simulink model "TST_DrvDem_SelectParameter"  (R2016b)
settings: Solver=FixedStepDiscrete  StartTime=0.0  StopTime=simTime  FixedStep=sampleTime  RelTol=1e-3
values from neighbouring files (symbols this model uses):
  testCase = 1    [initTST_DrvDem_SelectParameter_001.m]    (also in initTST_DrvDem_SelectParameter_002.m = 2; initTST_DrvDem_SelectParameter_003.m = 3)
libraries: simulink x82, UnitTest_Lib x78
(part 2 of 3)

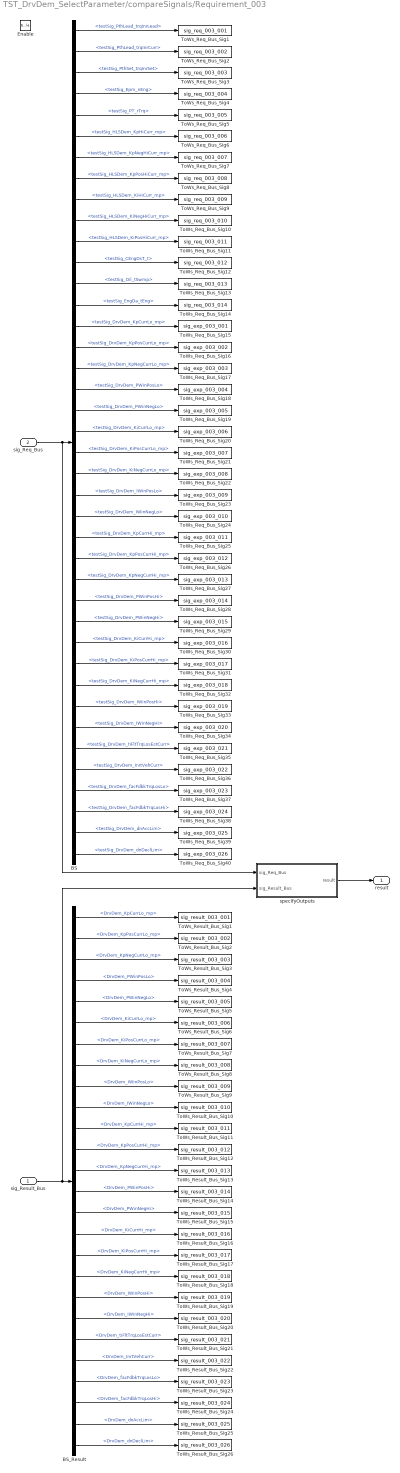
== system TST_DrvDem_SelectParameter/compareSignals/Requirement_003 ==
  sig_Result_Bus : Inport
  sig_Req_Bus : Inport  Port=2
  Enable : EnablePort
  BS : BusSelector  OutputSignals=testSig_PthLead_trqInrLead,testSig_PthLead_trqInrCurr,testSig_PthSet_trqInrSet,testSig_Epm_nEng,testSig_PT_rTrq,testSig_HLSDem_KpHiCurr_mp,testSig_HLSDem_KpNegHiCurr_mp,testSig_HLSDem_KpPosHiCurr_mp,testSig_HLSDem_KiHiCurr_mp,testSig_HLSDem_KiNegHiCurr_mp,testSig_HLSDem_KiPosHiCurr_mp,testSig_CEngDsT_t,testSig_Oil_tSwmp,testSig_EngDa_tEng,testSig_DrvDem_KpCurrLo_mp,testSig_DrvDem_KpPosCurrLo_mp,testSig_DrvDem_KpNegCurrLo_mp,testSig_DrvDem_PWinPosLo,testSig_DrvDem_PWinNegLo,testSig_DrvDem_KiCurrLo_mp,testSig_DrvDem_KiPosCurrLo_mp,testSig_DrvDem_KiNegCurrLo_mp,testSig_DrvDem_IWinPosLo,testSig_DrvDem_IWinNegLo,testSig_DrvDem_KpCurrHi_mp,testSig_DrvDem_KpPosCurrHi_mp,testSig_DrvDem_KpNegCurrHi_mp,testSig_DrvDem_PWinPosHi,testSig_DrvDem_PWinNegHi,testSig_DrvDem_KiCurrHi_mp,testSig_DrvDem_KiPosCurrHi_mp,testSig_DrvDem_KiNegCurrHi_mp,testSig_DrvDem_IWinPosHi,testSig_DrvDem_IWinNegHi,testSig_DrvDem_tiFltTrqLosEstCurr,testSig_DrvDem_InrtVehCurr,testSig_DrvDem_facFdbkTrqLosLo,testSig_DrvDem_facFdbkTrqLosHi,testSig_DrvDem_dnAccLim,testSig_DrvDem_dnDeclLim
  BS_Result : BusSelector  OutputSignals=DrvDem_KpCurrLo_mp,DrvDem_KpPosCurrLo_mp,DrvDem_KpNegCurrLo_mp,DrvDem_PWinPosLo,DrvDem_PWinNegLo,DrvDem_KiCurrLo_mp,DrvDem_KiPosCurrLo_mp,DrvDem_KiNegCurrLo_mp,DrvDem_IWinPosLo,DrvDem_IWinNegLo,DrvDem_KpCurrHi_mp,DrvDem_KpPosCurrHi_mp,DrvDem_KpNegCurrHi_mp,DrvDem_PWinPosHi,DrvDem_PWinNegHi,DrvDem_KiCurrHi_mp,DrvDem_KiPosCurrHi_mp,DrvDem_KiNegCurrHi_mp,DrvDem_IWinPosHi,DrvDem_IWinNegHi,DrvDem_tiFltTrqLosEstCurr,DrvDem_InrtVehCurr,DrvDem_facFdbkTrqLosLo,DrvDem_facFdbkTrqLosHi,DrvDem_dnAccLim,DrvDem_dnDeclLim
  ToWs_Req_Bus_Sig1 : ToWorkspace  VariableName=sig_req_003_001  SaveFormat=Structure With Time
  ToWs_Req_Bus_Sig10 : ToWorkspace  VariableName=sig_req_003_010  SaveFormat=Structure With Time
  ToWs_Req_Bus_Sig11 : ToWorkspace  VariableName=sig_req_003_011  SaveFormat=Structure With Time
  ToWs_Req_Bus_Sig12 : ToWorkspace  VariableName=sig_req_003_012  SaveFormat=Structure With Time
  ToWs_Req_Bus_Sig13 : ToWorkspace  VariableName=sig_req_003_013  SaveFormat=Structure With Time
  ToWs_Req_Bus_Sig14 : ToWorkspace  VariableName=sig_req_003_014  SaveFormat=Structure With Time
  ToWs_Req_Bus_Sig15 : ToWorkspace  VariableName=sig_exp_003_001  SaveFormat=Structure With Time
  ToWs_Req_Bus_Sig16 : ToWorkspace  VariableName=sig_exp_003_002  SaveFormat=Structure With Time
  ToWs_Req_Bus_Sig17 : ToWorkspace  VariableName=sig_exp_003_003  SaveFormat=Structure With Time
  ToWs_Req_Bus_Sig18 : ToWorkspace  VariableName=sig_exp_003_004  SaveFormat=Structure With Time
  ToWs_Req_Bus_Sig19 : ToWorkspace  VariableName=sig_exp_003_005  SaveFormat=Structure With Time
  ToWs_Req_Bus_Sig2 : ToWorkspace  VariableName=sig_req_003_002  SaveFormat=Structure With Time
  ToWs_Req_Bus_Sig20 : ToWorkspace  VariableName=sig_exp_003_006  SaveFormat=Structure With Time
  ToWs_Req_Bus_Sig21 : ToWorkspace  VariableName=sig_exp_003_007  SaveFormat=Structure With Time
  ToWs_Req_Bus_Sig22 : ToWorkspace  VariableName=sig_exp_003_008  SaveFormat=Structure With Time
  ToWs_Req_Bus_Sig23 : ToWorkspace  VariableName=sig_exp_003_009  SaveFormat=Structure With Time
  ToWs_Req_Bus_Sig24 : ToWorkspace  VariableName=sig_exp_003_010  SaveFormat=Structure With Time
  ToWs_Req_Bus_Sig25 : ToWorkspace  VariableName=sig_exp_003_011  SaveFormat=Structure With Time
  ToWs_Req_Bus_Sig26 : ToWorkspace  VariableName=sig_exp_003_012  SaveFormat=Structure With Time
  ToWs_Req_Bus_Sig27 : ToWorkspace  VariableName=sig_exp_003_013  SaveFormat=Structure With Time
  ToWs_Req_Bus_Sig28 : ToWorkspace  VariableName=sig_exp_003_014  SaveFormat=Structure With Time
  ToWs_Req_Bus_Sig29 : ToWorkspace  VariableName=sig_exp_003_015  SaveFormat=Structure With Time
  ToWs_Req_Bus_Sig3 : ToWorkspace  VariableName=sig_req_003_003  SaveFormat=Structure With Time
  ToWs_Req_Bus_Sig30 : ToWorkspace  VariableName=sig_exp_003_016  SaveFormat=Structure With Time
  ToWs_Req_Bus_Sig31 : ToWorkspace  VariableName=sig_exp_003_017  SaveFormat=Structure With Time
  ToWs_Req_Bus_Sig32 : ToWorkspace  VariableName=sig_exp_003_018  SaveFormat=Structure With Time
  ToWs_Req_Bus_Sig33 : ToWorkspace  VariableName=sig_exp_003_019  SaveFormat=Structure With Time
  ToWs_Req_Bus_Sig34 : ToWorkspace  VariableName=sig_exp_003_020  SaveFormat=Structure With Time
  ToWs_Req_Bus_Sig35 : ToWorkspace  VariableName=sig_exp_003_021  SaveFormat=Structure With Time
  ToWs_Req_Bus_Sig36 : ToWorkspace  VariableName=sig_exp_003_022  SaveFormat=Structure With Time
  ToWs_Req_Bus_Sig37 : ToWorkspace  VariableName=sig_exp_003_023  SaveFormat=Structure With Time
  ToWs_Req_Bus_Sig38 : ToWorkspace  VariableName=sig_exp_003_024  SaveFormat=Structure With Time
  ToWs_Req_Bus_Sig39 : ToWorkspace  VariableName=sig_exp_003_025  SaveFormat=Structure With Time
  ToWs_Req_Bus_Sig4 : ToWorkspace  VariableName=sig_req_003_004  SaveFormat=Structure With Time
  ToWs_Req_Bus_Sig40 : ToWorkspace  VariableName=sig_exp_003_026  SaveFormat=Structure With Time
  ToWs_Req_Bus_Sig5 : ToWorkspace  VariableName=sig_req_003_005  SaveFormat=Structure With Time
  ToWs_Req_Bus_Sig6 : ToWorkspace  VariableName=sig_req_003_006  SaveFormat=Structure With Time
  ToWs_Req_Bus_Sig7 : ToWorkspace  VariableName=sig_req_003_007  SaveFormat=Structure With Time
  ToWs_Req_Bus_Sig8 : ToWorkspace  VariableName=sig_req_003_008  SaveFormat=Structure With Time
  ToWs_Req_Bus_Sig9 : ToWorkspace  VariableName=sig_req_003_009  SaveFormat=Structure With Time
  ToWs_Result_Bus_Sig1 : ToWorkspace  VariableName=sig_result_003_001  SaveFormat=Structure With Time
  ToWs_Result_Bus_Sig10 : ToWorkspace  VariableName=sig_result_003_010  SaveFormat=Structure With Time
  ToWs_Result_Bus_Sig11 : ToWorkspace  VariableName=sig_result_003_011  SaveFormat=Structure With Time
  ToWs_Result_Bus_Sig12 : ToWorkspace  VariableName=sig_result_003_012  SaveFormat=Structure With Time
  ToWs_Result_Bus_Sig13 : ToWorkspace  VariableName=sig_result_003_013  SaveFormat=Structure With Time
  ToWs_Result_Bus_Sig14 : ToWorkspace  VariableName=sig_result_003_014  SaveFormat=Structure With Time
  ToWs_Result_Bus_Sig15 : ToWorkspace  VariableName=sig_result_003_015  SaveFormat=Structure With Time
  ToWs_Result_Bus_Sig16 : ToWorkspace  VariableName=sig_result_003_016  SaveFormat=Structure With Time
  ToWs_Result_Bus_Sig17 : ToWorkspace  VariableName=sig_result_003_017  SaveFormat=Structure With Time
  ToWs_Result_Bus_Sig18 : ToWorkspace  VariableName=sig_result_003_018  SaveFormat=Structure With Time
  ToWs_Result_Bus_Sig19 : ToWorkspace  VariableName=sig_result_003_019  SaveFormat=Structure With Time
  ToWs_Result_Bus_Sig2 : ToWorkspace  VariableName=sig_result_003_002  SaveFormat=Structure With Time
  ToWs_Result_Bus_Sig20 : ToWorkspace  VariableName=sig_result_003_020  SaveFormat=Structure With Time
  ToWs_Result_Bus_Sig21 : ToWorkspace  VariableName=sig_result_003_021  SaveFormat=Structure With Time
  ToWs_Result_Bus_Sig22 : ToWorkspace  VariableName=sig_result_003_022  SaveFormat=Structure With Time
  ToWs_Result_Bus_Sig23 : ToWorkspace  VariableName=sig_result_003_023  SaveFormat=Structure With Time
  ToWs_Result_Bus_Sig24 : ToWorkspace  VariableName=sig_result_003_024  SaveFormat=Structure With Time
  ToWs_Result_Bus_Sig25 : ToWorkspace  VariableName=sig_result_003_025  SaveFormat=Structure With Time
  ToWs_Result_Bus_Sig26 : ToWorkspace  VariableName=sig_result_003_026  SaveFormat=Structure With Time
  ToWs_Result_Bus_Sig3 : ToWorkspace  VariableName=sig_result_003_003  SaveFormat=Structure With Time
  ToWs_Result_Bus_Sig4 : ToWorkspace  VariableName=sig_result_003_004  SaveFormat=Structure With Time
  ToWs_Result_Bus_Sig5 : ToWorkspace  VariableName=sig_result_003_005  SaveFormat=Structure With Time
  ToWs_Result_Bus_Sig6 : ToWorkspace  VariableName=sig_result_003_006  SaveFormat=Structure With Time
  ToWs_Result_Bus_Sig7 : ToWorkspace  VariableName=sig_result_003_007  SaveFormat=Structure With Time
  ToWs_Result_Bus_Sig8 : ToWorkspace  VariableName=sig_result_003_008  SaveFormat=Structure With Time
  ToWs_Result_Bus_Sig9 : ToWorkspace  VariableName=sig_result_003_009  SaveFormat=Structure With Time
  specifyOutputs : Subsystem
  result : Outport
  wires:
  sig_Req_Bus/1 -> BS/1, specifyOutputs/1(sig_Req_Bus)
  BS/1 -> ToWs_Req_Bus_Sig1/1  "<testSig_PthLead_trqInrLead>"
  BS/2 -> ToWs_Req_Bus_Sig2/1  "<testSig_PthLead_trqInrCurr>"
  BS/3 -> ToWs_Req_Bus_Sig3/1  "<testSig_PthSet_trqInrSet>"
  BS/4 -> ToWs_Req_Bus_Sig4/1  "<testSig_Epm_nEng>"
  BS/5 -> ToWs_Req_Bus_Sig5/1  "<testSig_PT_rTrq>"
  BS/6 -> ToWs_Req_Bus_Sig6/1  "<testSig_HLSDem_KpHiCurr_mp>"
  BS/7 -> ToWs_Req_Bus_Sig7/1  "<testSig_HLSDem_KpNegHiCurr_mp>"
  BS/8 -> ToWs_Req_Bus_Sig8/1  "<testSig_HLSDem_KpPosHiCurr_mp>"
  BS/9 -> ToWs_Req_Bus_Sig9/1  "<testSig_HLSDem_KiHiCurr_mp>"
  BS/10 -> ToWs_Req_Bus_Sig10/1  "<testSig_HLSDem_KiNegHiCurr_mp>"
  BS/11 -> ToWs_Req_Bus_Sig11/1  "<testSig_HLSDem_KiPosHiCurr_mp>"
  BS/12 -> ToWs_Req_Bus_Sig12/1  "<testSig_CEngDsT_t>"
  BS/13 -> ToWs_Req_Bus_Sig13/1  "<testSig_Oil_tSwmp>"
  BS/14 -> ToWs_Req_Bus_Sig14/1  "<testSig_EngDa_tEng>"
  BS/15 -> ToWs_Req_Bus_Sig15/1  "<testSig_DrvDem_KpCurrLo_mp>"
  BS/16 -> ToWs_Req_Bus_Sig16/1  "<testSig_DrvDem_KpPosCurrLo_mp>"
  BS/17 -> ToWs_Req_Bus_Sig17/1  "<testSig_DrvDem_KpNegCurrLo_mp>"
  BS/18 -> ToWs_Req_Bus_Sig18/1  "<testSig_DrvDem_PWinPosLo>"
  BS/19 -> ToWs_Req_Bus_Sig19/1  "<testSig_DrvDem_PWinNegLo>"
  BS/20 -> ToWs_Req_Bus_Sig20/1  "<testSig_DrvDem_KiCurrLo_mp>"
  BS/21 -> ToWs_Req_Bus_Sig21/1  "<testSig_DrvDem_KiPosCurrLo_mp>"
  BS/22 -> ToWs_Req_Bus_Sig22/1  "<testSig_DrvDem_KiNegCurrLo_mp>"
  BS/23 -> ToWs_Req_Bus_Sig23/1  "<testSig_DrvDem_IWinPosLo>"
  BS/24 -> ToWs_Req_Bus_Sig24/1  "<testSig_DrvDem_IWinNegLo>"
  BS/25 -> ToWs_Req_Bus_Sig25/1  "<testSig_DrvDem_KpCurrHi_mp>"
  BS/26 -> ToWs_Req_Bus_Sig26/1  "<testSig_DrvDem_KpPosCurrHi_mp>"
  BS/27 -> ToWs_Req_Bus_Sig27/1  "<testSig_DrvDem_KpNegCurrHi_mp>"
  BS/28 -> ToWs_Req_Bus_Sig28/1  "<testSig_DrvDem_PWinPosHi>"
  BS/29 -> ToWs_Req_Bus_Sig29/1  "<testSig_DrvDem_PWinNegHi>"
  BS/30 -> ToWs_Req_Bus_Sig30/1  "<testSig_DrvDem_KiCurrHi_mp>"
  BS/31 -> ToWs_Req_Bus_Sig31/1  "<testSig_DrvDem_KiPosCurrHi_mp>"
  BS/32 -> ToWs_Req_Bus_Sig32/1  "<testSig_DrvDem_KiNegCurrHi_mp>"
  BS/33 -> ToWs_Req_Bus_Sig33/1  "<testSig_DrvDem_IWinPosHi>"
  BS/34 -> ToWs_Req_Bus_Sig34/1  "<testSig_DrvDem_IWinNegHi>"
  BS/35 -> ToWs_Req_Bus_Sig35/1  "<testSig_DrvDem_tiFltTrqLosEstCurr>"
  BS/36 -> ToWs_Req_Bus_Sig36/1  "<testSig_DrvDem_InrtVehCurr>"
  BS/37 -> ToWs_Req_Bus_Sig37/1  "<testSig_DrvDem_facFdbkTrqLosLo>"
  BS/38 -> ToWs_Req_Bus_Sig38/1  "<testSig_DrvDem_facFdbkTrqLosHi>"
  BS/39 -> ToWs_Req_Bus_Sig39/1  "<testSig_DrvDem_dnAccLim>"
  BS/40 -> ToWs_Req_Bus_Sig40/1  "<testSig_DrvDem_dnDeclLim>"
  sig_Result_Bus/1 -> BS_Result/1, specifyOutputs/2(sig_Result_Bus)
  BS_Result/1 -> ToWs_Result_Bus_Sig1/1  "<DrvDem_KpCurrLo_mp>"
  BS_Result/2 -> ToWs_Result_Bus_Sig2/1  "<DrvDem_KpPosCurrLo_mp>"
  BS_Result/3 -> ToWs_Result_Bus_Sig3/1  "<DrvDem_KpNegCurrLo_mp>"
  BS_Result/4 -> ToWs_Result_Bus_Sig4/1  "<DrvDem_PWinPosLo>"
  BS_Result/5 -> ToWs_Result_Bus_Sig5/1  "<DrvDem_PWinNegLo>"
  BS_Result/6 -> ToWs_Result_Bus_Sig6/1  "<DrvDem_KiCurrLo_mp>"
  BS_Result/7 -> ToWs_Result_Bus_Sig7/1  "<DrvDem_KiPosCurrLo_mp>"
  BS_Result/8 -> ToWs_Result_Bus_Sig8/1  "<DrvDem_KiNegCurrLo_mp>"
  BS_Result/9 -> ToWs_Result_Bus_Sig9/1  "<DrvDem_IWinPosLo>"
  BS_Result/10 -> ToWs_Result_Bus_Sig10/1  "<DrvDem_IWinNegLo>"
  BS_Result/11 -> ToWs_Result_Bus_Sig11/1  "<DrvDem_KpCurrHi_mp>"
  BS_Result/12 -> ToWs_Result_Bus_Sig12/1  "<DrvDem_KpPosCurrHi_mp>"
  BS_Result/13 -> ToWs_Result_Bus_Sig13/1  "<DrvDem_KpNegCurrHi_mp>"
  BS_Result/14 -> ToWs_Result_Bus_Sig14/1  "<DrvDem_PWinPosHi>"
  BS_Result/15 -> ToWs_Result_Bus_Sig15/1  "<DrvDem_PWinNegHi>"
  BS_Result/16 -> ToWs_Result_Bus_Sig16/1  "<DrvDem_KiCurrHi_mp>"
  BS_Result/17 -> ToWs_Result_Bus_Sig17/1  "<DrvDem_KiPosCurrHi_mp>"
  BS_Result/18 -> ToWs_Result_Bus_Sig18/1  "<DrvDem_KiNegCurrHi_mp>"
  BS_Result/19 -> ToWs_Result_Bus_Sig19/1  "<DrvDem_IWinPosHi>"
  BS_Result/20 -> ToWs_Result_Bus_Sig20/1  "<DrvDem_IWinNegHi>"
  BS_Result/21 -> ToWs_Result_Bus_Sig21/1  "<DrvDem_tiFltTrqLosEstCurr>"
  BS_Result/22 -> ToWs_Result_Bus_Sig22/1  "<DrvDem_InrtVehCurr>"
  BS_Result/23 -> ToWs_Result_Bus_Sig23/1  "<DrvDem_facFdbkTrqLosLo>"
  BS_Result/24 -> ToWs_Result_Bus_Sig24/1  "<DrvDem_facFdbkTrqLosHi>"
  BS_Result/25 -> ToWs_Result_Bus_Sig25/1  "<DrvDem_dnAccLim>"
  BS_Result/26 -> ToWs_Result_Bus_Sig26/1  "<DrvDem_dnDeclLim>"
  specifyOutputs/1(result) -> result/1

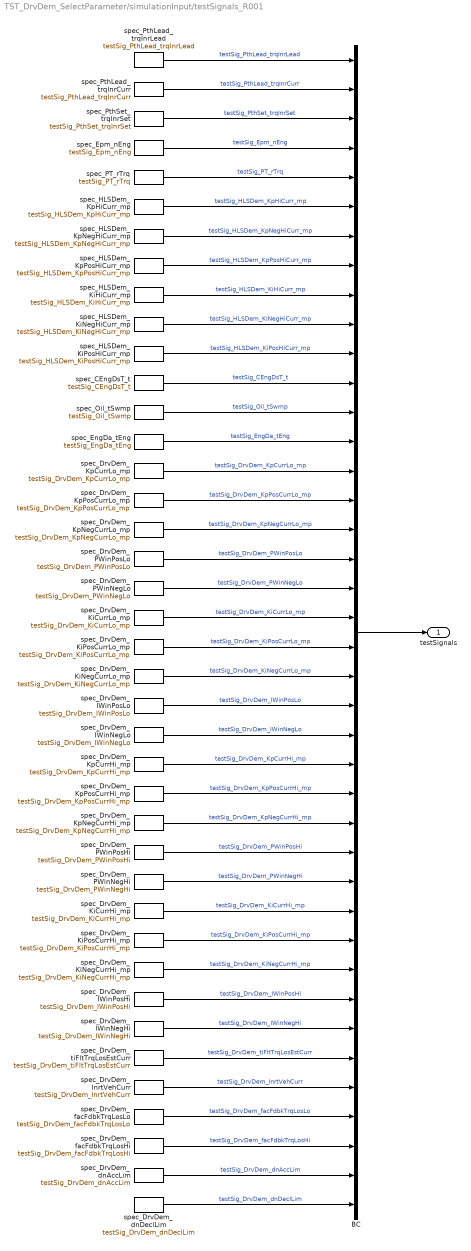
== system TST_DrvDem_SelectParameter/simulationInput/testSignals_R001 ==
  BC : BusCreator  Inputs=40
  spec_CEngDsT_t : FromWorkspace  VariableName=testSig_CEngDsT_t  Interpolate=off  OutputAfterFinalValue=Holding final value
  spec_DrvDem_IWinNegHi : FromWorkspace  VariableName=testSig_DrvDem_IWinNegHi  Interpolate=off  OutputAfterFinalValue=Holding final value
  spec_DrvDem_IWinNegLo : FromWorkspace  VariableName=testSig_DrvDem_IWinNegLo  Interpolate=off  OutputAfterFinalValue=Holding final value
  spec_DrvDem_IWinPosHi : FromWorkspace  VariableName=testSig_DrvDem_IWinPosHi  Interpolate=off  OutputAfterFinalValue=Holding final value
  spec_DrvDem_IWinPosLo : FromWorkspace  VariableName=testSig_DrvDem_IWinPosLo  Interpolate=off  OutputAfterFinalValue=Holding final value
  spec_DrvDem_InrtVehCurr : FromWorkspace  VariableName=testSig_DrvDem_InrtVehCurr  Interpolate=off  OutputAfterFinalValue=Holding final value
  spec_DrvDem_KiCurrHi_mp : FromWorkspace  VariableName=testSig_DrvDem_KiCurrHi_mp  Interpolate=off  OutputAfterFinalValue=Holding final value
  spec_DrvDem_KiCurrLo_mp : FromWorkspace  VariableName=testSig_DrvDem_KiCurrLo_mp  Interpolate=off  OutputAfterFinalValue=Holding final value
  spec_DrvDem_KiNegCurrHi_mp : FromWorkspace  VariableName=testSig_DrvDem_KiNegCurrHi_mp  Interpolate=off  OutputAfterFinalValue=Holding final value
  spec_DrvDem_KiNegCurrLo_mp : FromWorkspace  VariableName=testSig_DrvDem_KiNegCurrLo_mp  Interpolate=off  OutputAfterFinalValue=Holding final value
  spec_DrvDem_KiPosCurrHi_mp : FromWorkspace  VariableName=testSig_DrvDem_KiPosCurrHi_mp  Interpolate=off  OutputAfterFinalValue=Holding final value
  spec_DrvDem_KiPosCurrLo_mp : FromWorkspace  VariableName=testSig_DrvDem_KiPosCurrLo_mp  Interpolate=off  OutputAfterFinalValue=Holding final value
  spec_DrvDem_KpCurrHi_mp : FromWorkspace  VariableName=testSig_DrvDem_KpCurrHi_mp  Interpolate=off  OutputAfterFinalValue=Holding final value
  spec_DrvDem_KpCurrLo_mp : FromWorkspace  VariableName=testSig_DrvDem_KpCurrLo_mp  Interpolate=off  OutputAfterFinalValue=Holding final value
  spec_DrvDem_KpNegCurrHi_mp : FromWorkspace  VariableName=testSig_DrvDem_KpNegCurrHi_mp  Interpolate=off  OutputAfterFinalValue=Holding final value
  spec_DrvDem_KpNegCurrLo_mp : FromWorkspace  VariableName=testSig_DrvDem_KpNegCurrLo_mp  Interpolate=off  OutputAfterFinalValue=Holding final value
  spec_DrvDem_KpPosCurrHi_mp : FromWorkspace  VariableName=testSig_DrvDem_KpPosCurrHi_mp  Interpolate=off  OutputAfterFinalValue=Holding final value
  spec_DrvDem_KpPosCurrLo_mp : FromWorkspace  VariableName=testSig_DrvDem_KpPosCurrLo_mp  Interpolate=off  OutputAfterFinalValue=Holding final value
  spec_DrvDem_PWinNegHi : FromWorkspace  VariableName=testSig_DrvDem_PWinNegHi  Interpolate=off  OutputAfterFinalValue=Holding final value
  spec_DrvDem_PWinNegLo : FromWorkspace  VariableName=testSig_DrvDem_PWinNegLo  Interpolate=off  OutputAfterFinalValue=Holding final value
  spec_DrvDem_PWinPosHi : FromWorkspace  VariableName=testSig_DrvDem_PWinPosHi  Interpolate=off  OutputAfterFinalValue=Holding final value
  spec_DrvDem_PWinPosLo : FromWorkspace  VariableName=testSig_DrvDem_PWinPosLo  Interpolate=off  OutputAfterFinalValue=Holding final value
  spec_DrvDem_dnAccLim : FromWorkspace  VariableName=testSig_DrvDem_dnAccLim  Interpolate=off  OutputAfterFinalValue=Holding final value
  spec_DrvDem_dnDeclLim : FromWorkspace  VariableName=testSig_DrvDem_dnDeclLim  Interpolate=off  OutputAfterFinalValue=Holding final value
  spec_DrvDem_facFdbkTrqLosHi : FromWorkspace  VariableName=testSig_DrvDem_facFdbkTrqLosHi  Interpolate=off  OutputAfterFinalValue=Holding final value
  spec_DrvDem_facFdbkTrqLosLo : FromWorkspace  VariableName=testSig_DrvDem_facFdbkTrqLosLo  Interpolate=off  OutputAfterFinalValue=Holding final value
  spec_DrvDem_tiFltTrqLosEstCurr : FromWorkspace  VariableName=testSig_DrvDem_tiFltTrqLosEstCurr  Interpolate=off  OutputAfterFinalValue=Holding final value
  spec_EngDa_tEng : FromWorkspace  VariableName=testSig_EngDa_tEng  Interpolate=off  OutputAfterFinalValue=Holding final value
  spec_Epm_nEng : FromWorkspace  VariableName=testSig_Epm_nEng  Interpolate=off  OutputAfterFinalValue=Holding final value
  spec_HLSDem_KiHiCurr_mp : FromWorkspace  VariableName=testSig_HLSDem_KiHiCurr_mp  Interpolate=off  OutputAfterFinalValue=Holding final value
  spec_HLSDem_KiNegHiCurr_mp : FromWorkspace  VariableName=testSig_HLSDem_KiNegHiCurr_mp  Interpolate=off  OutputAfterFinalValue=Holding final value
  spec_HLSDem_KiPosHiCurr_mp : FromWorkspace  VariableName=testSig_HLSDem_KiPosHiCurr_mp  Interpolate=off  OutputAfterFinalValue=Holding final value
  spec_HLSDem_KpHiCurr_mp : FromWorkspace  VariableName=testSig_HLSDem_KpHiCurr_mp  Interpolate=off  OutputAfterFinalValue=Holding final value
  spec_HLSDem_KpNegHiCurr_mp : FromWorkspace  VariableName=testSig_HLSDem_KpNegHiCurr_mp  Interpolate=off  OutputAfterFinalValue=Holding final value
  spec_HLSDem_KpPosHiCurr_mp : FromWorkspace  VariableName=testSig_HLSDem_KpPosHiCurr_mp  Interpolate=off  OutputAfterFinalValue=Holding final value
  spec_Oil_tSwmp : FromWorkspace  VariableName=testSig_Oil_tSwmp  Interpolate=off  OutputAfterFinalValue=Holding final value
  spec_PT_rTrq : FromWorkspace  VariableName=testSig_PT_rTrq  Interpolate=off  OutputAfterFinalValue=Holding final value
  spec_PthLead_trqInrCurr : FromWorkspace  VariableName=testSig_PthLead_trqInrCurr  Interpolate=off  OutputAfterFinalValue=Holding final value
  spec_PthLead_trqInrLead : FromWorkspace  VariableName=testSig_PthLead_trqInrLead  Interpolate=off  OutputAfterFinalValue=Holding final value
  spec_PthSet_trqInrSet : FromWorkspace  VariableName=testSig_PthSet_trqInrSet  Interpolate=off  OutputAfterFinalValue=Holding final value
  testSignals : Outport
  wires:
  BC/1 -> testSignals/1
  spec_PthLead_trqInrLead/1 -> BC/1  "testSig_PthLead_trqInrLead"
  spec_PthLead_trqInrCurr/1 -> BC/2  "testSig_PthLead_trqInrCurr"
  spec_PthSet_trqInrSet/1 -> BC/3  "testSig_PthSet_trqInrSet"
  spec_Epm_nEng/1 -> BC/4  "testSig_Epm_nEng"
  spec_PT_rTrq/1 -> BC/5  "testSig_PT_rTrq"
  spec_HLSDem_KpHiCurr_mp/1 -> BC/6  "testSig_HLSDem_KpHiCurr_mp"
  spec_HLSDem_KpNegHiCurr_mp/1 -> BC/7  "testSig_HLSDem_KpNegHiCurr_mp"
  spec_HLSDem_KpPosHiCurr_mp/1 -> BC/8  "testSig_HLSDem_KpPosHiCurr_mp"
  spec_HLSDem_KiHiCurr_mp/1 -> BC/9  "testSig_HLSDem_KiHiCurr_mp"
  spec_HLSDem_KiNegHiCurr_mp/1 -> BC/10  "testSig_HLSDem_KiNegHiCurr_mp"
  spec_HLSDem_KiPosHiCurr_mp/1 -> BC/11  "testSig_HLSDem_KiPosHiCurr_mp"
  spec_CEngDsT_t/1 -> BC/12  "testSig_CEngDsT_t"
  spec_Oil_tSwmp/1 -> BC/13  "testSig_Oil_tSwmp"
  spec_EngDa_tEng/1 -> BC/14  "testSig_EngDa_tEng"
  spec_DrvDem_KpCurrLo_mp/1 -> BC/15  "testSig_DrvDem_KpCurrLo_mp"
  spec_DrvDem_KpPosCurrLo_mp/1 -> BC/16  "testSig_DrvDem_KpPosCurrLo_mp"
  spec_DrvDem_KpNegCurrLo_mp/1 -> BC/17  "testSig_DrvDem_KpNegCurrLo_mp"
  spec_DrvDem_PWinPosLo/1 -> BC/18  "testSig_DrvDem_PWinPosLo"
  spec_DrvDem_PWinNegLo/1 -> BC/19  "testSig_DrvDem_PWinNegLo"
  spec_DrvDem_KiCurrLo_mp/1 -> BC/20  "testSig_DrvDem_KiCurrLo_mp"
  spec_DrvDem_KiPosCurrLo_mp/1 -> BC/21  "testSig_DrvDem_KiPosCurrLo_mp"
  spec_DrvDem_KiNegCurrLo_mp/1 -> BC/22  "testSig_DrvDem_KiNegCurrLo_mp"
  spec_DrvDem_IWinPosLo/1 -> BC/23  "testSig_DrvDem_IWinPosLo"
  spec_DrvDem_IWinNegLo/1 -> BC/24  "testSig_DrvDem_IWinNegLo"
  spec_DrvDem_KpCurrHi_mp/1 -> BC/25  "testSig_DrvDem_KpCurrHi_mp"
  spec_DrvDem_KpPosCurrHi_mp/1 -> BC/26  "testSig_DrvDem_KpPosCurrHi_mp"
  spec_DrvDem_KpNegCurrHi_mp/1 -> BC/27  "testSig_DrvDem_KpNegCurrHi_mp"
  spec_DrvDem_PWinPosHi/1 -> BC/28  "testSig_DrvDem_PWinPosHi"
  spec_DrvDem_PWinNegHi/1 -> BC/29  "testSig_DrvDem_PWinNegHi"
  spec_DrvDem_KiCurrHi_mp/1 -> BC/30  "testSig_DrvDem_KiCurrHi_mp"
  spec_DrvDem_KiPosCurrHi_mp/1 -> BC/31  "testSig_DrvDem_KiPosCurrHi_mp"
  spec_DrvDem_KiNegCurrHi_mp/1 -> BC/32  "testSig_DrvDem_KiNegCurrHi_mp"
  spec_DrvDem_IWinPosHi/1 -> BC/33  "testSig_DrvDem_IWinPosHi"
  spec_DrvDem_IWinNegHi/1 -> BC/34  "testSig_DrvDem_IWinNegHi"
  spec_DrvDem_tiFltTrqLosEstCurr/1 -> BC/35  "testSig_DrvDem_tiFltTrqLosEstCurr"
  spec_DrvDem_InrtVehCurr/1 -> BC/36  "testSig_DrvDem_InrtVehCurr"
  spec_DrvDem_facFdbkTrqLosLo/1 -> BC/37  "testSig_DrvDem_facFdbkTrqLosLo"
  spec_DrvDem_facFdbkTrqLosHi/1 -> BC/38  "testSig_DrvDem_facFdbkTrqLosHi"
  spec_DrvDem_dnAccLim/1 -> BC/39  "testSig_DrvDem_dnAccLim"
  spec_DrvDem_dnDeclLim/1 -> BC/40  "testSig_DrvDem_dnDeclLim"

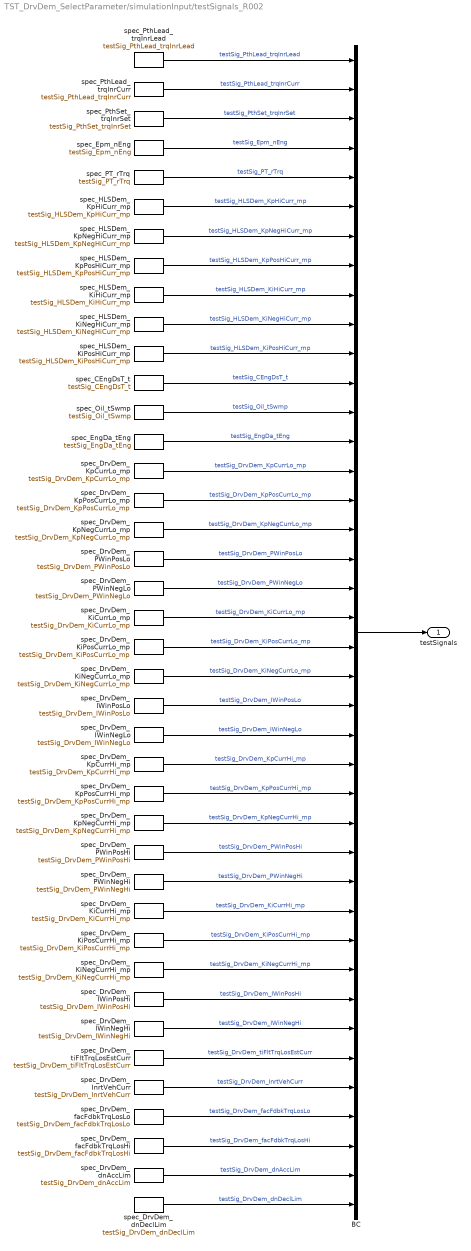
== system TST_DrvDem_SelectParameter/simulationInput/testSignals_R002 ==
  BC : BusCreator  Inputs=40
  spec_CEngDsT_t : FromWorkspace  VariableName=testSig_CEngDsT_t  Interpolate=off  OutputAfterFinalValue=Holding final value
  spec_DrvDem_IWinNegHi : FromWorkspace  VariableName=testSig_DrvDem_IWinNegHi  Interpolate=off  OutputAfterFinalValue=Holding final value
  spec_DrvDem_IWinNegLo : FromWorkspace  VariableName=testSig_DrvDem_IWinNegLo  Interpolate=off  OutputAfterFinalValue=Holding final value
  spec_DrvDem_IWinPosHi : FromWorkspace  VariableName=testSig_DrvDem_IWinPosHi  Interpolate=off  OutputAfterFinalValue=Holding final value
  spec_DrvDem_IWinPosLo : FromWorkspace  VariableName=testSig_DrvDem_IWinPosLo  Interpolate=off  OutputAfterFinalValue=Holding final value
  spec_DrvDem_InrtVehCurr : FromWorkspace  VariableName=testSig_DrvDem_InrtVehCurr  Interpolate=off  OutputAfterFinalValue=Holding final value
  spec_DrvDem_KiCurrHi_mp : FromWorkspace  VariableName=testSig_DrvDem_KiCurrHi_mp  Interpolate=off  OutputAfterFinalValue=Holding final value
  spec_DrvDem_KiCurrLo_mp : FromWorkspace  VariableName=testSig_DrvDem_KiCurrLo_mp  Interpolate=off  OutputAfterFinalValue=Holding final value
  spec_DrvDem_KiNegCurrHi_mp : FromWorkspace  VariableName=testSig_DrvDem_KiNegCurrHi_mp  Interpolate=off  OutputAfterFinalValue=Holding final value
  spec_DrvDem_KiNegCurrLo_mp : FromWorkspace  VariableName=testSig_DrvDem_KiNegCurrLo_mp  Interpolate=off  OutputAfterFinalValue=Holding final value
  spec_DrvDem_KiPosCurrHi_mp : FromWorkspace  VariableName=testSig_DrvDem_KiPosCurrHi_mp  Interpolate=off  OutputAfterFinalValue=Holding final value
  spec_DrvDem_KiPosCurrLo_mp : FromWorkspace  VariableName=testSig_DrvDem_KiPosCurrLo_mp  Interpolate=off  OutputAfterFinalValue=Holding final value
  spec_DrvDem_KpCurrHi_mp : FromWorkspace  VariableName=testSig_DrvDem_KpCurrHi_mp  Interpolate=off  OutputAfterFinalValue=Holding final value
  spec_DrvDem_KpCurrLo_mp : FromWorkspace  VariableName=testSig_DrvDem_KpCurrLo_mp  Interpolate=off  OutputAfterFinalValue=Holding final value
  spec_DrvDem_KpNegCurrHi_mp : FromWorkspace  VariableName=testSig_DrvDem_KpNegCurrHi_mp  Interpolate=off  OutputAfterFinalValue=Holding final value
  spec_DrvDem_KpNegCurrLo_mp : FromWorkspace  VariableName=testSig_DrvDem_KpNegCurrLo_mp  Interpolate=off  OutputAfterFinalValue=Holding final value
  spec_DrvDem_KpPosCurrHi_mp : FromWorkspace  VariableName=testSig_DrvDem_KpPosCurrHi_mp  Interpolate=off  OutputAfterFinalValue=Holding final value
  spec_DrvDem_KpPosCurrLo_mp : FromWorkspace  VariableName=testSig_DrvDem_KpPosCurrLo_mp  Interpolate=off  OutputAfterFinalValue=Holding final value
  spec_DrvDem_PWinNegHi : FromWorkspace  VariableName=testSig_DrvDem_PWinNegHi  Interpolate=off  OutputAfterFinalValue=Holding final value
  spec_DrvDem_PWinNegLo : FromWorkspace  VariableName=testSig_DrvDem_PWinNegLo  Interpolate=off  OutputAfterFinalValue=Holding final value
  spec_DrvDem_PWinPosHi : FromWorkspace  VariableName=testSig_DrvDem_PWinPosHi  Interpolate=off  OutputAfterFinalValue=Holding final value
  spec_DrvDem_PWinPosLo : FromWorkspace  VariableName=testSig_DrvDem_PWinPosLo  Interpolate=off  OutputAfterFinalValue=Holding final value
  spec_DrvDem_dnAccLim : FromWorkspace  VariableName=testSig_DrvDem_dnAccLim  Interpolate=off  OutputAfterFinalValue=Holding final value
  spec_DrvDem_dnDeclLim : FromWorkspace  VariableName=testSig_DrvDem_dnDeclLim  Interpolate=off  OutputAfterFinalValue=Holding final value
  spec_DrvDem_facFdbkTrqLosHi : FromWorkspace  VariableName=testSig_DrvDem_facFdbkTrqLosHi  Interpolate=off  OutputAfterFinalValue=Holding final value
  spec_DrvDem_facFdbkTrqLosLo : FromWorkspace  VariableName=testSig_DrvDem_facFdbkTrqLosLo  Interpolate=off  OutputAfterFinalValue=Holding final value
  spec_DrvDem_tiFltTrqLosEstCurr : FromWorkspace  VariableName=testSig_DrvDem_tiFltTrqLosEstCurr  Interpolate=off  OutputAfterFinalValue=Holding final value
  spec_EngDa_tEng : FromWorkspace  VariableName=testSig_EngDa_tEng  Interpolate=off  OutputAfterFinalValue=Holding final value
  spec_Epm_nEng : FromWorkspace  VariableName=testSig_Epm_nEng  Interpolate=off  OutputAfterFinalValue=Holding final value
  spec_HLSDem_KiHiCurr_mp : FromWorkspace  VariableName=testSig_HLSDem_KiHiCurr_mp  Interpolate=off  OutputAfterFinalValue=Holding final value
  spec_HLSDem_KiNegHiCurr_mp : FromWorkspace  VariableName=testSig_HLSDem_KiNegHiCurr_mp  Interpolate=off  OutputAfterFinalValue=Holding final value
  spec_HLSDem_KiPosHiCurr_mp : FromWorkspace  VariableName=testSig_HLSDem_KiPosHiCurr_mp  Interpolate=off  OutputAfterFinalValue=Holding final value
  spec_HLSDem_KpHiCurr_mp : FromWorkspace  VariableName=testSig_HLSDem_KpHiCurr_mp  Interpolate=off  OutputAfterFinalValue=Holding final value
  spec_HLSDem_KpNegHiCurr_mp : FromWorkspace  VariableName=testSig_HLSDem_KpNegHiCurr_mp  Interpolate=off  OutputAfterFinalValue=Holding final value
  spec_HLSDem_KpPosHiCurr_mp : FromWorkspace  VariableName=testSig_HLSDem_KpPosHiCurr_mp  Interpolate=off  OutputAfterFinalValue=Holding final value
  spec_Oil_tSwmp : FromWorkspace  VariableName=testSig_Oil_tSwmp  Interpolate=off  OutputAfterFinalValue=Holding final value
  spec_PT_rTrq : FromWorkspace  VariableName=testSig_PT_rTrq  Interpolate=off  OutputAfterFinalValue=Holding final value
  spec_PthLead_trqInrCurr : FromWorkspace  VariableName=testSig_PthLead_trqInrCurr  Interpolate=off  OutputAfterFinalValue=Holding final value
  spec_PthLead_trqInrLead : FromWorkspace  VariableName=testSig_PthLead_trqInrLead  Interpolate=off  OutputAfterFinalValue=Holding final value
  spec_PthSet_trqInrSet : FromWorkspace  VariableName=testSig_PthSet_trqInrSet  Interpolate=off  OutputAfterFinalValue=Holding final value
  testSignals : Outport
  wires:
  BC/1 -> testSignals/1
  spec_PthLead_trqInrLead/1 -> BC/1  "testSig_PthLead_trqInrLead"
  spec_PthLead_trqInrCurr/1 -> BC/2  "testSig_PthLead_trqInrCurr"
  spec_PthSet_trqInrSet/1 -> BC/3  "testSig_PthSet_trqInrSet"
  spec_Epm_nEng/1 -> BC/4  "testSig_Epm_nEng"
  spec_PT_rTrq/1 -> BC/5  "testSig_PT_rTrq"
  spec_HLSDem_KpHiCurr_mp/1 -> BC/6  "testSig_HLSDem_KpHiCurr_mp"
  spec_HLSDem_KpNegHiCurr_mp/1 -> BC/7  "testSig_HLSDem_KpNegHiCurr_mp"
  spec_HLSDem_KpPosHiCurr_mp/1 -> BC/8  "testSig_HLSDem_KpPosHiCurr_mp"
  spec_HLSDem_KiHiCurr_mp/1 -> BC/9  "testSig_HLSDem_KiHiCurr_mp"
  spec_HLSDem_KiNegHiCurr_mp/1 -> BC/10  "testSig_HLSDem_KiNegHiCurr_mp"
  spec_HLSDem_KiPosHiCurr_mp/1 -> BC/11  "testSig_HLSDem_KiPosHiCurr_mp"
  spec_CEngDsT_t/1 -> BC/12  "testSig_CEngDsT_t"
  spec_Oil_tSwmp/1 -> BC/13  "testSig_Oil_tSwmp"
  spec_EngDa_tEng/1 -> BC/14  "testSig_EngDa_tEng"
  spec_DrvDem_KpCurrLo_mp/1 -> BC/15  "testSig_DrvDem_KpCurrLo_mp"
  spec_DrvDem_KpPosCurrLo_mp/1 -> BC/16  "testSig_DrvDem_KpPosCurrLo_mp"
  spec_DrvDem_KpNegCurrLo_mp/1 -> BC/17  "testSig_DrvDem_KpNegCurrLo_mp"
  spec_DrvDem_PWinPosLo/1 -> BC/18  "testSig_DrvDem_PWinPosLo"
  spec_DrvDem_PWinNegLo/1 -> BC/19  "testSig_DrvDem_PWinNegLo"
  spec_DrvDem_KiCurrLo_mp/1 -> BC/20  "testSig_DrvDem_KiCurrLo_mp"
  spec_DrvDem_KiPosCurrLo_mp/1 -> BC/21  "testSig_DrvDem_KiPosCurrLo_mp"
  spec_DrvDem_KiNegCurrLo_mp/1 -> BC/22  "testSig_DrvDem_KiNegCurrLo_mp"
  spec_DrvDem_IWinPosLo/1 -> BC/23  "testSig_DrvDem_IWinPosLo"
  spec_DrvDem_IWinNegLo/1 -> BC/24  "testSig_DrvDem_IWinNegLo"
  spec_DrvDem_KpCurrHi_mp/1 -> BC/25  "testSig_DrvDem_KpCurrHi_mp"
  spec_DrvDem_KpPosCurrHi_mp/1 -> BC/26  "testSig_DrvDem_KpPosCurrHi_mp"
  spec_DrvDem_KpNegCurrHi_mp/1 -> BC/27  "testSig_DrvDem_KpNegCurrHi_mp"
  spec_DrvDem_PWinPosHi/1 -> BC/28  "testSig_DrvDem_PWinPosHi"
  spec_DrvDem_PWinNegHi/1 -> BC/29  "testSig_DrvDem_PWinNegHi"
  spec_DrvDem_KiCurrHi_mp/1 -> BC/30  "testSig_DrvDem_KiCurrHi_mp"
  spec_DrvDem_KiPosCurrHi_mp/1 -> BC/31  "testSig_DrvDem_KiPosCurrHi_mp"
  spec_DrvDem_KiNegCurrHi_mp/1 -> BC/32  "testSig_DrvDem_KiNegCurrHi_mp"
  spec_DrvDem_IWinPosHi/1 -> BC/33  "testSig_DrvDem_IWinPosHi"
  spec_DrvDem_IWinNegHi/1 -> BC/34  "testSig_DrvDem_IWinNegHi"
  spec_DrvDem_tiFltTrqLosEstCurr/1 -> BC/35  "testSig_DrvDem_tiFltTrqLosEstCurr"
  spec_DrvDem_InrtVehCurr/1 -> BC/36  "testSig_DrvDem_InrtVehCurr"
  spec_DrvDem_facFdbkTrqLosLo/1 -> BC/37  "testSig_DrvDem_facFdbkTrqLosLo"
  spec_DrvDem_facFdbkTrqLosHi/1 -> BC/38  "testSig_DrvDem_facFdbkTrqLosHi"
  spec_DrvDem_dnAccLim/1 -> BC/39  "testSig_DrvDem_dnAccLim"
  spec_DrvDem_dnDeclLim/1 -> BC/40  "testSig_DrvDem_dnDeclLim"

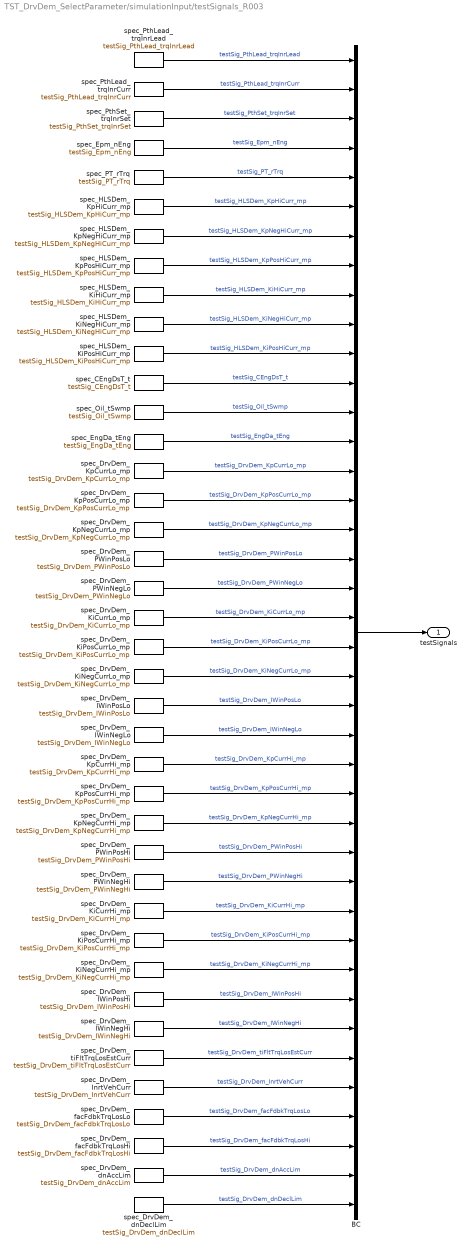
== system TST_DrvDem_SelectParameter/simulationInput/testSignals_R003 ==
  BC : BusCreator  Inputs=40
  spec_CEngDsT_t : FromWorkspace  VariableName=testSig_CEngDsT_t  Interpolate=off  OutputAfterFinalValue=Holding final value
  spec_DrvDem_IWinNegHi : FromWorkspace  VariableName=testSig_DrvDem_IWinNegHi  Interpolate=off  OutputAfterFinalValue=Holding final value
  spec_DrvDem_IWinNegLo : FromWorkspace  VariableName=testSig_DrvDem_IWinNegLo  Interpolate=off  OutputAfterFinalValue=Holding final value
  spec_DrvDem_IWinPosHi : FromWorkspace  VariableName=testSig_DrvDem_IWinPosHi  Interpolate=off  OutputAfterFinalValue=Holding final value
  spec_DrvDem_IWinPosLo : FromWorkspace  VariableName=testSig_DrvDem_IWinPosLo  Interpolate=off  OutputAfterFinalValue=Holding final value
  spec_DrvDem_InrtVehCurr : FromWorkspace  VariableName=testSig_DrvDem_InrtVehCurr  Interpolate=off  OutputAfterFinalValue=Holding final value
  spec_DrvDem_KiCurrHi_mp : FromWorkspace  VariableName=testSig_DrvDem_KiCurrHi_mp  Interpolate=off  OutputAfterFinalValue=Holding final value
  spec_DrvDem_KiCurrLo_mp : FromWorkspace  VariableName=testSig_DrvDem_KiCurrLo_mp  Interpolate=off  OutputAfterFinalValue=Holding final value
  spec_DrvDem_KiNegCurrHi_mp : FromWorkspace  VariableName=testSig_DrvDem_KiNegCurrHi_mp  Interpolate=off  OutputAfterFinalValue=Holding final value
  spec_DrvDem_KiNegCurrLo_mp : FromWorkspace  VariableName=testSig_DrvDem_KiNegCurrLo_mp  Interpolate=off  OutputAfterFinalValue=Holding final value
  spec_DrvDem_KiPosCurrHi_mp : FromWorkspace  VariableName=testSig_DrvDem_KiPosCurrHi_mp  Interpolate=off  OutputAfterFinalValue=Holding final value
  spec_DrvDem_KiPosCurrLo_mp : FromWorkspace  VariableName=testSig_DrvDem_KiPosCurrLo_mp  Interpolate=off  OutputAfterFinalValue=Holding final value
  spec_DrvDem_KpCurrHi_mp : FromWorkspace  VariableName=testSig_DrvDem_KpCurrHi_mp  Interpolate=off  OutputAfterFinalValue=Holding final value
  spec_DrvDem_KpCurrLo_mp : FromWorkspace  VariableName=testSig_DrvDem_KpCurrLo_mp  Interpolate=off  OutputAfterFinalValue=Holding final value
  spec_DrvDem_KpNegCurrHi_mp : FromWorkspace  VariableName=testSig_DrvDem_KpNegCurrHi_mp  Interpolate=off  OutputAfterFinalValue=Holding final value
  spec_DrvDem_KpNegCurrLo_mp : FromWorkspace  VariableName=testSig_DrvDem_KpNegCurrLo_mp  Interpolate=off  OutputAfterFinalValue=Holding final value
  spec_DrvDem_KpPosCurrHi_mp : FromWorkspace  VariableName=testSig_DrvDem_KpPosCurrHi_mp  Interpolate=off  OutputAfterFinalValue=Holding final value
  spec_DrvDem_KpPosCurrLo_mp : FromWorkspace  VariableName=testSig_DrvDem_KpPosCurrLo_mp  Interpolate=off  OutputAfterFinalValue=Holding final value
  spec_DrvDem_PWinNegHi : FromWorkspace  VariableName=testSig_DrvDem_PWinNegHi  Interpolate=off  OutputAfterFinalValue=Holding final value
  spec_DrvDem_PWinNegLo : FromWorkspace  VariableName=testSig_DrvDem_PWinNegLo  Interpolate=off  OutputAfterFinalValue=Holding final value
  spec_DrvDem_PWinPosHi : FromWorkspace  VariableName=testSig_DrvDem_PWinPosHi  Interpolate=off  OutputAfterFinalValue=Holding final value
  spec_DrvDem_PWinPosLo : FromWorkspace  VariableName=testSig_DrvDem_PWinPosLo  Interpolate=off  OutputAfterFinalValue=Holding final value
  spec_DrvDem_dnAccLim : FromWorkspace  VariableName=testSig_DrvDem_dnAccLim  Interpolate=off  OutputAfterFinalValue=Holding final value
  spec_DrvDem_dnDeclLim : FromWorkspace  VariableName=testSig_DrvDem_dnDeclLim  Interpolate=off  OutputAfterFinalValue=Holding final value
  spec_DrvDem_facFdbkTrqLosHi : FromWorkspace  VariableName=testSig_DrvDem_facFdbkTrqLosHi  Interpolate=off  OutputAfterFinalValue=Holding final value
  spec_DrvDem_facFdbkTrqLosLo : FromWorkspace  VariableName=testSig_DrvDem_facFdbkTrqLosLo  Interpolate=off  OutputAfterFinalValue=Holding final value
  spec_DrvDem_tiFltTrqLosEstCurr : FromWorkspace  VariableName=testSig_DrvDem_tiFltTrqLosEstCurr  Interpolate=off  OutputAfterFinalValue=Holding final value
  spec_EngDa_tEng : FromWorkspace  VariableName=testSig_EngDa_tEng  Interpolate=off  OutputAfterFinalValue=Holding final value
  spec_Epm_nEng : FromWorkspace  VariableName=testSig_Epm_nEng  Interpolate=off  OutputAfterFinalValue=Holding final value
  spec_HLSDem_KiHiCurr_mp : FromWorkspace  VariableName=testSig_HLSDem_KiHiCurr_mp  Interpolate=off  OutputAfterFinalValue=Holding final value
  spec_HLSDem_KiNegHiCurr_mp : FromWorkspace  VariableName=testSig_HLSDem_KiNegHiCurr_mp  Interpolate=off  OutputAfterFinalValue=Holding final value
  spec_HLSDem_KiPosHiCurr_mp : FromWorkspace  VariableName=testSig_HLSDem_KiPosHiCurr_mp  Interpolate=off  OutputAfterFinalValue=Holding final value
  spec_HLSDem_KpHiCurr_mp : FromWorkspace  VariableName=testSig_HLSDem_KpHiCurr_mp  Interpolate=off  OutputAfterFinalValue=Holding final value
  spec_HLSDem_KpNegHiCurr_mp : FromWorkspace  VariableName=testSig_HLSDem_KpNegHiCurr_mp  Interpolate=off  OutputAfterFinalValue=Holding final value
  spec_HLSDem_KpPosHiCurr_mp : FromWorkspace  VariableName=testSig_HLSDem_KpPosHiCurr_mp  Interpolate=off  OutputAfterFinalValue=Holding final value
  spec_Oil_tSwmp : FromWorkspace  VariableName=testSig_Oil_tSwmp  Interpolate=off  OutputAfterFinalValue=Holding final value
  spec_PT_rTrq : FromWorkspace  VariableName=testSig_PT_rTrq  Interpolate=off  OutputAfterFinalValue=Holding final value
  spec_PthLead_trqInrCurr : FromWorkspace  VariableName=testSig_PthLead_trqInrCurr  Interpolate=off  OutputAfterFinalValue=Holding final value
  spec_PthLead_trqInrLead : FromWorkspace  VariableName=testSig_PthLead_trqInrLead  Interpolate=off  OutputAfterFinalValue=Holding final value
  spec_PthSet_trqInrSet : FromWorkspace  VariableName=testSig_PthSet_trqInrSet  Interpolate=off  OutputAfterFinalValue=Holding final value
  testSignals : Outport
  wires:
  BC/1 -> testSignals/1
  spec_PthLead_trqInrLead/1 -> BC/1  "testSig_PthLead_trqInrLead"
  spec_PthLead_trqInrCurr/1 -> BC/2  "testSig_PthLead_trqInrCurr"
  spec_PthSet_trqInrSet/1 -> BC/3  "testSig_PthSet_trqInrSet"
  spec_Epm_nEng/1 -> BC/4  "testSig_Epm_nEng"
  spec_PT_rTrq/1 -> BC/5  "testSig_PT_rTrq"
  spec_HLSDem_KpHiCurr_mp/1 -> BC/6  "testSig_HLSDem_KpHiCurr_mp"
  spec_HLSDem_KpNegHiCurr_mp/1 -> BC/7  "testSig_HLSDem_KpNegHiCurr_mp"
  spec_HLSDem_KpPosHiCurr_mp/1 -> BC/8  "testSig_HLSDem_KpPosHiCurr_mp"
  spec_HLSDem_KiHiCurr_mp/1 -> BC/9  "testSig_HLSDem_KiHiCurr_mp"
  spec_HLSDem_KiNegHiCurr_mp/1 -> BC/10  "testSig_HLSDem_KiNegHiCurr_mp"
  spec_HLSDem_KiPosHiCurr_mp/1 -> BC/11  "testSig_HLSDem_KiPosHiCurr_mp"
  spec_CEngDsT_t/1 -> BC/12  "testSig_CEngDsT_t"
  spec_Oil_tSwmp/1 -> BC/13  "testSig_Oil_tSwmp"
  spec_EngDa_tEng/1 -> BC/14  "testSig_EngDa_tEng"
  spec_DrvDem_KpCurrLo_mp/1 -> BC/15  "testSig_DrvDem_KpCurrLo_mp"
  spec_DrvDem_KpPosCurrLo_mp/1 -> BC/16  "testSig_DrvDem_KpPosCurrLo_mp"
  spec_DrvDem_KpNegCurrLo_mp/1 -> BC/17  "testSig_DrvDem_KpNegCurrLo_mp"
  spec_DrvDem_PWinPosLo/1 -> BC/18  "testSig_DrvDem_PWinPosLo"
  spec_DrvDem_PWinNegLo/1 -> BC/19  "testSig_DrvDem_PWinNegLo"
  spec_DrvDem_KiCurrLo_mp/1 -> BC/20  "testSig_DrvDem_KiCurrLo_mp"
  spec_DrvDem_KiPosCurrLo_mp/1 -> BC/21  "testSig_DrvDem_KiPosCurrLo_mp"
  spec_DrvDem_KiNegCurrLo_mp/1 -> BC/22  "testSig_DrvDem_KiNegCurrLo_mp"
  spec_DrvDem_IWinPosLo/1 -> BC/23  "testSig_DrvDem_IWinPosLo"
  spec_DrvDem_IWinNegLo/1 -> BC/24  "testSig_DrvDem_IWinNegLo"
  spec_DrvDem_KpCurrHi_mp/1 -> BC/25  "testSig_DrvDem_KpCurrHi_mp"
  spec_DrvDem_KpPosCurrHi_mp/1 -> BC/26  "testSig_DrvDem_KpPosCurrHi_mp"
  spec_DrvDem_KpNegCurrHi_mp/1 -> BC/27  "testSig_DrvDem_KpNegCurrHi_mp"
  spec_DrvDem_PWinPosHi/1 -> BC/28  "testSig_DrvDem_PWinPosHi"
  spec_DrvDem_PWinNegHi/1 -> BC/29  "testSig_DrvDem_PWinNegHi"
  spec_DrvDem_KiCurrHi_mp/1 -> BC/30  "testSig_DrvDem_KiCurrHi_mp"
  spec_DrvDem_KiPosCurrHi_mp/1 -> BC/31  "testSig_DrvDem_KiPosCurrHi_mp"
  spec_DrvDem_KiNegCurrHi_mp/1 -> BC/32  "testSig_DrvDem_KiNegCurrHi_mp"
  spec_DrvDem_IWinPosHi/1 -> BC/33  "testSig_DrvDem_IWinPosHi"
  spec_DrvDem_IWinNegHi/1 -> BC/34  "testSig_DrvDem_IWinNegHi"
  spec_DrvDem_tiFltTrqLosEstCurr/1 -> BC/35  "testSig_DrvDem_tiFltTrqLosEstCurr"
  spec_DrvDem_InrtVehCurr/1 -> BC/36  "testSig_DrvDem_InrtVehCurr"
  spec_DrvDem_facFdbkTrqLosLo/1 -> BC/37  "testSig_DrvDem_facFdbkTrqLosLo"
  spec_DrvDem_facFdbkTrqLosHi/1 -> BC/38  "testSig_DrvDem_facFdbkTrqLosHi"
  spec_DrvDem_dnAccLim/1 -> BC/39  "testSig_DrvDem_dnAccLim"
  spec_DrvDem_dnDeclLim/1 -> BC/40  "testSig_DrvDem_dnDeclLim"

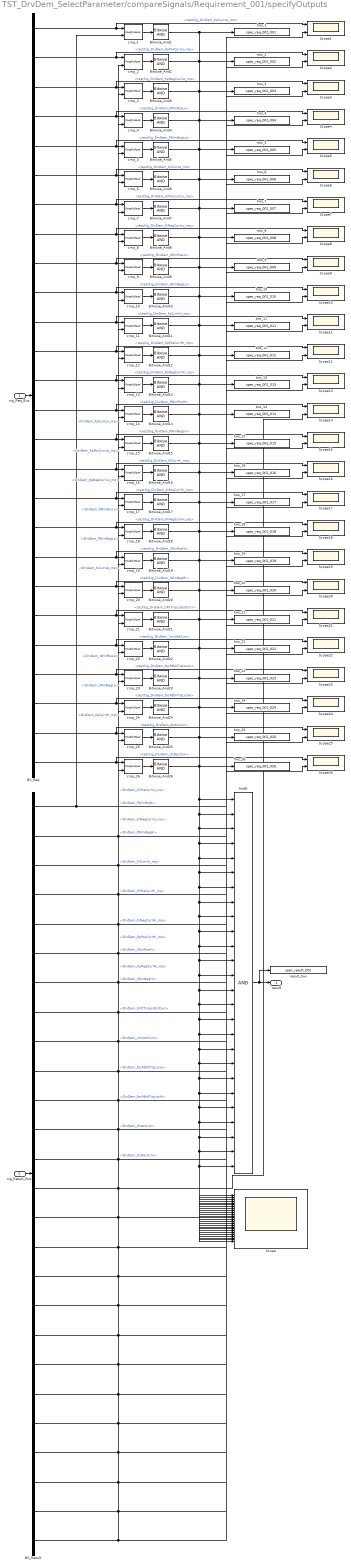
== system TST_DrvDem_SelectParameter/compareSignals/Requirement_001/specifyOutputs ==
  sig_Req_Bus : Inport
  sig_Result_Bus : Inport  Port=2
  AndN : Logic  Inputs=26
  BS_Req : BusSelector  OutputSignals=testSig_DrvDem_KpCurrLo_mp,testSig_DrvDem_KpPosCurrLo_mp,testSig_DrvDem_KpNegCurrLo_mp,testSig_DrvDem_PWinPosLo,testSig_DrvDem_PWinNegLo,testSig_DrvDem_KiCurrLo_mp,testSig_DrvDem_KiPosCurrLo_mp,testSig_DrvDem_KiNegCurrLo_mp,testSig_DrvDem_IWinPosLo,testSig_DrvDem_IWinNegLo,testSig_DrvDem_KpCurrHi_mp,testSig_DrvDem_KpPosCurrHi_mp,testSig_DrvDem_KpNegCurrHi_mp,testSig_DrvDem_PWinPosHi,testSig_DrvDem_PWinNegHi,testSig_DrvDem_KiCurrHi_mp,testSig_DrvDem_KiPosCurrHi_mp,testSig_DrvDem_KiNegCurrHi_mp,testSig_DrvDem_IWinPosHi,testSig_DrvDem_IWinNegHi,testSig_DrvDem_tiFltTrqLosEstCurr,testSig_DrvDem_InrtVehCurr,testSig_DrvDem_facFdbkTrqLosLo,testSig_DrvDem_facFdbkTrqLosHi,testSig_DrvDem_dnAccLim,testSig_DrvDem_dnDeclLim
  BS_Result : BusSelector  OutputSignals=DrvDem_KpCurrLo_mp,DrvDem_KpPosCurrLo_mp,DrvDem_KpNegCurrLo_mp,DrvDem_PWinPosLo,DrvDem_PWinNegLo,DrvDem_KiCurrLo_mp,DrvDem_KiPosCurrLo_mp,DrvDem_KiNegCurrLo_mp,DrvDem_IWinPosLo,DrvDem_IWinNegLo,DrvDem_KpCurrHi_mp,DrvDem_KpPosCurrHi_mp,DrvDem_KpNegCurrHi_mp,DrvDem_PWinPosHi,DrvDem_PWinNegHi,DrvDem_KiCurrHi_mp,DrvDem_KiPosCurrHi_mp,DrvDem_KiNegCurrHi_mp,DrvDem_IWinPosHi,DrvDem_IWinNegHi,DrvDem_tiFltTrqLosEstCurr,DrvDem_InrtVehCurr,DrvDem_facFdbkTrqLosLo,DrvDem_facFdbkTrqLosHi,DrvDem_dnAccLim,DrvDem_dnDeclLim
  Bitwise_And{1..26} (26 alike) : simulink/Logic and Bit Operations/Bitwise Operator  logicop=AND  UseBitMask=off  BitMask=bin2dec('11011001')  BitMaskRealWorld=Stored Integer
  Scope : Scope  NumInputPorts=26
  Scope{1..26} (26 alike) : Scope  NumInputPorts=2
  cmp_{1..24} (24 alike) : UnitTest_Lib/RoughlyEqual  slope=0.1
  cmp_25 : UnitTest_Lib/RoughlyEqual  slope=1
  cmp_26 : UnitTest_Lib/RoughlyEqual  slope=1
  result_tws : ToWorkspace  VariableName=spec_result_001
  tws_1 : ToWorkspace  VariableName=spec_req_001_001
  tws_10 : ToWorkspace  VariableName=spec_req_001_010
  tws_11 : ToWorkspace  VariableName=spec_req_001_011
  tws_12 : ToWorkspace  VariableName=spec_req_001_012
  tws_13 : ToWorkspace  VariableName=spec_req_001_013
  tws_14 : ToWorkspace  VariableName=spec_req_001_014
  tws_15 : ToWorkspace  VariableName=spec_req_001_015
  tws_16 : ToWorkspace  VariableName=spec_req_001_016
  tws_17 : ToWorkspace  VariableName=spec_req_001_017
  tws_18 : ToWorkspace  VariableName=spec_req_001_018
  tws_19 : ToWorkspace  VariableName=spec_req_001_019
  tws_2 : ToWorkspace  VariableName=spec_req_001_002
  tws_20 : ToWorkspace  VariableName=spec_req_001_020
  tws_21 : ToWorkspace  VariableName=spec_req_001_021
  tws_22 : ToWorkspace  VariableName=spec_req_001_022
  tws_23 : ToWorkspace  VariableName=spec_req_001_023
  tws_24 : ToWorkspace  VariableName=spec_req_001_024
  tws_25 : ToWorkspace  VariableName=spec_req_001_025
  tws_26 : ToWorkspace  VariableName=spec_req_001_026
  tws_3 : ToWorkspace  VariableName=spec_req_001_003
  tws_4 : ToWorkspace  VariableName=spec_req_001_004
  tws_5 : ToWorkspace  VariableName=spec_req_001_005
  tws_6 : ToWorkspace  VariableName=spec_req_001_006
  tws_7 : ToWorkspace  VariableName=spec_req_001_007
  tws_8 : ToWorkspace  VariableName=spec_req_001_008
  tws_9 : ToWorkspace  VariableName=spec_req_001_009
  result : Outport
  wires:
  sig_Req_Bus/1 -> BS_Req/1
  sig_Result_Bus/1 -> BS_Result/1
  AndN/1 -> result/1, result_tws/1
  BS_Req/1 -> cmp_1/1, Scope1/1  "<testSig_DrvDem_KpCurrLo_mp>"
  BS_Result/1 -> cmp_1/2, Scope1/2  "<DrvDem_KpCurrLo_mp>"
  cmp_1/1 -> Bitwise_And1/1
  Bitwise_And1/1 -> AndN/1, Scope/1, tws_1/1
  BS_Req/2 -> cmp_2/1, Scope2/1  "<testSig_DrvDem_KpPosCurrLo_mp>"
  BS_Result/2 -> cmp_2/2, Scope2/2  "<DrvDem_KpPosCurrLo_mp>"
  cmp_2/1 -> Bitwise_And2/1
  Bitwise_And2/1 -> AndN/2, Scope/2, tws_2/1
  BS_Req/3 -> cmp_3/1, Scope3/1  "<testSig_DrvDem_KpNegCurrLo_mp>"
  BS_Result/3 -> cmp_3/2, Scope3/2  "<DrvDem_KpNegCurrLo_mp>"
  cmp_3/1 -> Bitwise_And3/1
  Bitwise_And3/1 -> AndN/3, Scope/3, tws_3/1
  BS_Req/4 -> cmp_4/1, Scope4/1  "<testSig_DrvDem_PWinPosLo>"
  BS_Result/4 -> cmp_4/2, Scope4/2  "<DrvDem_PWinPosLo>"
  cmp_4/1 -> Bitwise_And4/1
  Bitwise_And4/1 -> AndN/4, Scope/4, tws_4/1
  BS_Req/5 -> cmp_5/1, Scope5/1  "<testSig_DrvDem_PWinNegLo>"
  BS_Result/5 -> cmp_5/2, Scope5/2  "<DrvDem_PWinNegLo>"
  cmp_5/1 -> Bitwise_And5/1
  Bitwise_And5/1 -> AndN/5, Scope/5, tws_5/1
  BS_Req/6 -> cmp_6/1, Scope6/1  "<testSig_DrvDem_KiCurrLo_mp>"
  BS_Result/6 -> cmp_6/2, Scope6/2  "<DrvDem_KiCurrLo_mp>"
  cmp_6/1 -> Bitwise_And6/1
  Bitwise_And6/1 -> AndN/6, Scope/6, tws_6/1
  BS_Req/7 -> cmp_7/1, Scope7/1  "<testSig_DrvDem_KiPosCurrLo_mp>"
  BS_Result/7 -> cmp_7/2, Scope7/2  "<DrvDem_KiPosCurrLo_mp>"
  cmp_7/1 -> Bitwise_And7/1
  Bitwise_And7/1 -> AndN/7, Scope/7, tws_7/1
  BS_Req/8 -> cmp_8/1, Scope8/1  "<testSig_DrvDem_KiNegCurrLo_mp>"
  BS_Result/8 -> cmp_8/2, Scope8/2  "<DrvDem_KiNegCurrLo_mp>"
  cmp_8/1 -> Bitwise_And8/1
  Bitwise_And8/1 -> AndN/8, Scope/8, tws_8/1
  BS_Req/9 -> cmp_9/1, Scope9/1  "<testSig_DrvDem_IWinPosLo>"
  BS_Result/9 -> cmp_9/2, Scope9/2  "<DrvDem_IWinPosLo>"
  cmp_9/1 -> Bitwise_And9/1
  Bitwise_And9/1 -> AndN/9, Scope/9, tws_9/1
  BS_Req/10 -> cmp_10/1, Scope10/1  "<testSig_DrvDem_IWinNegLo>"
  BS_Result/10 -> cmp_10/2, Scope10/2  "<DrvDem_IWinNegLo>"
  cmp_10/1 -> Bitwise_And10/1
  Bitwise_And10/1 -> AndN/10, Scope/10, tws_10/1
  BS_Req/11 -> cmp_11/1, Scope11/1  "<testSig_DrvDem_KpCurrHi_mp>"
  BS_Result/11 -> cmp_11/2, Scope11/2  "<DrvDem_KpCurrHi_mp>"
  cmp_11/1 -> Bitwise_And11/1
  Bitwise_And11/1 -> AndN/11, Scope/11, tws_11/1
  BS_Req/12 -> cmp_12/1, Scope12/1  "<testSig_DrvDem_KpPosCurrHi_mp>"
  BS_Result/12 -> cmp_12/2, Scope12/2  "<DrvDem_KpPosCurrHi_mp>"
  cmp_12/1 -> Bitwise_And12/1
  Bitwise_And12/1 -> AndN/12, Scope/12, tws_12/1
  BS_Req/13 -> cmp_13/1, Scope13/1  "<testSig_DrvDem_KpNegCurrHi_mp>"
  BS_Result/13 -> cmp_13/2, Scope13/2  "<DrvDem_KpNegCurrHi_mp>"
  cmp_13/1 -> Bitwise_And13/1
  Bitwise_And13/1 -> AndN/13, Scope/13, tws_13/1
  BS_Req/14 -> cmp_14/1, Scope14/1  "<testSig_DrvDem_PWinPosHi>"
  BS_Result/14 -> cmp_14/2, Scope14/2  "<DrvDem_PWinPosHi>"
  cmp_14/1 -> Bitwise_And14/1
  Bitwise_And14/1 -> AndN/14, Scope/14, tws_14/1
  BS_Req/15 -> cmp_15/1, Scope15/1  "<testSig_DrvDem_PWinNegHi>"
  BS_Result/15 -> cmp_15/2, Scope15/2  "<DrvDem_PWinNegHi>"
  cmp_15/1 -> Bitwise_And15/1
  Bitwise_And15/1 -> AndN/15, Scope/15, tws_15/1
  BS_Req/16 -> cmp_16/1, Scope16/1  "<testSig_DrvDem_KiCurrHi_mp>"
  BS_Result/16 -> cmp_16/2, Scope16/2  "<DrvDem_KiCurrHi_mp>"
  cmp_16/1 -> Bitwise_And16/1
  Bitwise_And16/1 -> AndN/16, Scope/16, tws_16/1
  BS_Req/17 -> cmp_17/1, Scope17/1  "<testSig_DrvDem_KiPosCurrHi_mp>"
  BS_Result/17 -> cmp_17/2, Scope17/2  "<DrvDem_KiPosCurrHi_mp>"
  cmp_17/1 -> Bitwise_And17/1
  Bitwise_And17/1 -> AndN/17, Scope/17, tws_17/1
  BS_Req/18 -> cmp_18/1, Scope18/1  "<testSig_DrvDem_KiNegCurrHi_mp>"
  BS_Result/18 -> cmp_18/2, Scope18/2  "<DrvDem_KiNegCurrHi_mp>"
  cmp_18/1 -> Bitwise_And18/1
  Bitwise_And18/1 -> AndN/18, Scope/18, tws_18/1
  BS_Req/19 -> cmp_19/1, Scope19/1  "<testSig_DrvDem_IWinPosHi>"
  BS_Result/19 -> cmp_19/2, Scope19/2  "<DrvDem_IWinPosHi>"
  cmp_19/1 -> Bitwise_And19/1
  Bitwise_And19/1 -> AndN/19, Scope/19, tws_19/1
  BS_Req/20 -> cmp_20/1, Scope20/1  "<testSig_DrvDem_IWinNegHi>"
  BS_Result/20 -> cmp_20/2, Scope20/2  "<DrvDem_IWinNegHi>"
  cmp_20/1 -> Bitwise_And20/1
  Bitwise_And20/1 -> AndN/20, Scope/20, tws_20/1
  BS_Req/21 -> cmp_21/1, Scope21/1  "<testSig_DrvDem_tiFltTrqLosEstCurr>"
  BS_Result/21 -> cmp_21/2, Scope21/2  "<DrvDem_tiFltTrqLosEstCurr>"
  cmp_21/1 -> Bitwise_And21/1
  Bitwise_And21/1 -> AndN/21, Scope/21, tws_21/1
  BS_Req/22 -> cmp_22/1, Scope22/1  "<testSig_DrvDem_InrtVehCurr>"
  BS_Result/22 -> cmp_22/2, Scope22/2  "<DrvDem_InrtVehCurr>"
  cmp_22/1 -> Bitwise_And22/1
  Bitwise_And22/1 -> AndN/22, Scope/22, tws_22/1
  BS_Req/23 -> cmp_23/1, Scope23/1  "<testSig_DrvDem_facFdbkTrqLosLo>"
  BS_Result/23 -> cmp_23/2, Scope23/2  "<DrvDem_facFdbkTrqLosLo>"
  cmp_23/1 -> Bitwise_And23/1
  Bitwise_And23/1 -> AndN/23, Scope/23, tws_23/1
  BS_Req/24 -> cmp_24/1, Scope24/1  "<testSig_DrvDem_facFdbkTrqLosHi>"
  BS_Result/24 -> cmp_24/2, Scope24/2  "<DrvDem_facFdbkTrqLosHi>"
  cmp_24/1 -> Bitwise_And24/1
  Bitwise_And24/1 -> AndN/24, Scope/24, tws_24/1
  BS_Req/25 -> cmp_25/1, Scope25/1  "<testSig_DrvDem_dnAccLim>"
  BS_Result/25 -> cmp_25/2, Scope25/2  "<DrvDem_dnAccLim>"
  cmp_25/1 -> Bitwise_And25/1
  Bitwise_And25/1 -> AndN/25, Scope/25, tws_25/1
  BS_Req/26 -> cmp_26/1, Scope26/1  "<testSig_DrvDem_dnDeclLim>"
  BS_Result/26 -> cmp_26/2, Scope26/2  "<DrvDem_dnDeclLim>"
  cmp_26/1 -> Bitwise_And26/1
  Bitwise_And26/1 -> AndN/26, Scope/26, tws_26/1
